simulink model "Controlled_simulink_model_vectorized"  (R2017b)
settings: Solver=VariableStepAuto  StartTime=0  StopTime=57  FixedStep=0.001  MaxStep=1e-4  MinStep=1e-5  RelTol=1e-5
values from neighbouring files (symbols this model uses):
  Accel_bias = 0    [Controlled_model_vectorized.m]
  Ax = 0.0    (= 0)    [Controlled_model_vectorized.m]
  Ay = 0.0    (= 0)    [Controlled_model_vectorized.m]
  Az = 0.0    (= 0)    [Controlled_model_vectorized.m]
  b = 1.144e-08    [Controlled_model_vectorized.m]
  b_m = 2.415e-6    (= 2.415e-06)    [Controlled_model_vectorized.m]
  d = 9.94e-10    [Controlled_model_vectorized.m]
  g = 9.81    [Controlled_model_vectorized.m]
  Gyro_bias = 0    [Controlled_model_vectorized.m]
  Ixx = 7.5*10^(-3)    (= 0.0075)    [Controlled_model_vectorized.m]
  Iyy = 7.5*10^(-3)    (= 0.0075)    [Controlled_model_vectorized.m]
  Izz = 1.3*10^(-2)    (= 0.013)    [Controlled_model_vectorized.m]
  Jr = 6.5*10^(-7)    (= 6.5e-07)    [Controlled_model_vectorized.m]
  Kemf = 0.00255    [Controlled_model_vectorized.m]
  Kt = Kemf    (= 0.00255)    [Controlled_model_vectorized.m]
  l = 0.23    [Controlled_model_vectorized.m]
  L = 0.001*R    (= 0.000117)    [Controlled_model_vectorized.m]
  m = weight/g    (= 0.0289500509684)    [Controlled_model_vectorized.m]
  R = 0.117    [Controlled_model_vectorized.m]
undefined symbols (not defined in the file or in its folder): sigbuilder_block
libraries: simulink x4
settings Model: Creator=Nicky  LastModifiedBy=Nicky
settings SolverCC: MaxConsecutiveMinStep=1000  ZeroCrossAlgorithm=Adaptive  AlgebraicLoopSolver=LineSearch  AutoInsertRateTranBlk=on
settings DebuggingCC: MaxConsecutiveZCsMsg=none
settings CodeAppCC: StateflowObjectComments=on
settings SimscapeCC: SimscapeNormalizeSystem=off

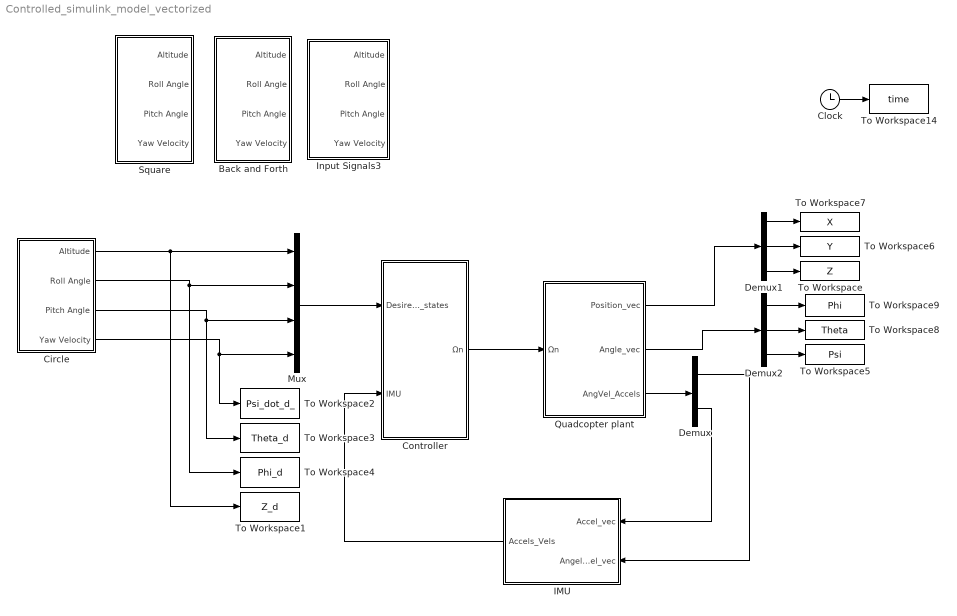
== system Controlled_simulink_model_vectorized ==
  Back and Forth : Subsystem  Tag=STV Subsys  LoadFcn=sigbuilder_block('load');  StartFcn=sigbuilder_block('start');  StopFcn=sigbuilder_block('stop');  ClipboardFcn=sigbuilder_block('clipboard');  mask(Sigbuilder block){tuvar=[0:10]}
      mask help: Simulink:masks:SigbuilderBlock_MD
      mask init:
      | if ~strcmp(get_param(bdroot(gcbh),'SimulationStatus'),'stopped') tuvar = sigbuilder_block('maskInit'); end
      settings: CopyFcn=sigbuilder_block('copy');  DeleteFcn=sigbuilder_block('delete');  ModelCloseFcn=sigbuilder_block('modelClose');  PreSaveFcn=sigbuilder_block('preSave');  PauseFcn=sigbuilder_block('pause');  ContinueFcn=sigbuilder_block('continue');  NameChangeFcn=sigbuilder_block('namechange');  OpenFcn=sigbuilder_block('open',[6 30 1428 682.5 ]);  CloseFcn=sigbuilder_block('close');
      mask Display: plot(0, 0, 100, 100,[2, 2, 32, 32, 2], [68, 8, 8, 68, 68],[32, 2], [38, 38], [32, 19, 2],[53, 60, 44], [32, 17, 17, 2],[16, 16, 31, 31]);txt = getActiveGroup(gcbh);text(2, 100, txt,'verticalAlignment', 'top');
  Circle : Subsystem  Tag=STV Subsys  LoadFcn=sigbuilder_block('load');  StartFcn=sigbuilder_block('start');  StopFcn=sigbuilder_block('stop');  ClipboardFcn=sigbuilder_block('clipboard');  mask(Sigbuilder block){tuvar=[0:10]}
      mask help: Simulink:masks:SigbuilderBlock_MD
      mask init:
      | if ~strcmp(get_param(bdroot(gcbh),'SimulationStatus'),'stopped') tuvar = sigbuilder_block('maskInit'); end
      settings: CopyFcn=sigbuilder_block('copy');  DeleteFcn=sigbuilder_block('delete');  ModelCloseFcn=sigbuilder_block('modelClose');  PreSaveFcn=sigbuilder_block('preSave');  PauseFcn=sigbuilder_block('pause');  ContinueFcn=sigbuilder_block('continue');  NameChangeFcn=sigbuilder_block('namechange');  OpenFcn=sigbuilder_block('open',[173.25 183.75 1012.5 456 ]);  CloseFcn=sigbuilder_block('close');
      mask Display: plot(0, 0, 100, 100,[2, 2, 32, 32, 2], [68, 8, 8, 68, 68],[32, 2], [38, 38], [32, 19, 2],[53, 60, 44], [32, 17, 17, 2],[16, 16, 31, 31]);txt = getActiveGroup(gcbh);text(2, 100, txt,'verticalAlignment', 'top');
  Clock : Clock
  Controller : Subsystem
  Demux : Demux  Outputs=2
  Demux1 : Demux  Outputs=3
  Demux2 : Demux  Outputs=3
  IMU : Subsystem
  Input Signals3 : Subsystem  Tag=STV Subsys  LoadFcn=sigbuilder_block('load');  StartFcn=sigbuilder_block('start');  StopFcn=sigbuilder_block('stop');  ClipboardFcn=sigbuilder_block('clipboard');  mask(Sigbuilder block){tuvar=[0:10]}
      mask help: Simulink:masks:SigbuilderBlock_MD
      mask init:
      | if ~strcmp(get_param(bdroot(gcbh),'SimulationStatus'),'stopped') tuvar = sigbuilder_block('maskInit'); end
      settings: CopyFcn=sigbuilder_block('copy');  DeleteFcn=sigbuilder_block('delete');  ModelCloseFcn=sigbuilder_block('modelClose');  PreSaveFcn=sigbuilder_block('preSave');  PauseFcn=sigbuilder_block('pause');  ContinueFcn=sigbuilder_block('continue');  NameChangeFcn=sigbuilder_block('namechange');  OpenFcn=sigbuilder_block('open',[6 46.5 1428 642 ]);  CloseFcn=sigbuilder_block('close');
      mask Display: plot(0, 0, 100, 100,[2, 2, 32, 32, 2], [68, 8, 8, 68, 68],[32, 2], [38, 38], [32, 19, 2],[53, 60, 44], [32, 17, 17, 2],[16, 16, 31, 31]);txt = getActiveGroup(gcbh);text(2, 100, txt,'verticalAlignment', 'top');
  Mux : Mux
  Quadcopter plant : Subsystem
  Square : Subsystem  Tag=STV Subsys  LoadFcn=sigbuilder_block('load');  StartFcn=sigbuilder_block('start');  StopFcn=sigbuilder_block('stop');  ClipboardFcn=sigbuilder_block('clipboard');  mask(Sigbuilder block){tuvar=[0:10]}
      mask help: Simulink:masks:SigbuilderBlock_MD
      mask init:
      | if ~strcmp(get_param(bdroot(gcbh),'SimulationStatus'),'stopped') tuvar = sigbuilder_block('maskInit'); end
      settings: CopyFcn=sigbuilder_block('copy');  DeleteFcn=sigbuilder_block('delete');  ModelCloseFcn=sigbuilder_block('modelClose');  PreSaveFcn=sigbuilder_block('preSave');  PauseFcn=sigbuilder_block('pause');  ContinueFcn=sigbuilder_block('continue');  NameChangeFcn=sigbuilder_block('namechange');  OpenFcn=sigbuilder_block('open',[6 30 1428 682.5 ]);  CloseFcn=sigbuilder_block('close');
      mask Display: plot(0, 0, 100, 100,[2, 2, 32, 32, 2], [68, 8, 8, 68, 68],[32, 2], [38, 38], [32, 19, 2],[53, 60, 44], [32, 17, 17, 2],[16, 16, 31, 31]);txt = getActiveGroup(gcbh);text(2, 100, txt,'verticalAlignment', 'top');
  To Workspace : ToWorkspace  VariableName=Z  SampleTime=0.001
      settings: Save2DSignal=2-D array (concatenate along first dimension)
  To Workspace1 : ToWorkspace  VariableName=Z_d  SampleTime=0.001
      settings: Save2DSignal=2-D array (concatenate along first dimension)
  To Workspace14 : ToWorkspace  VariableName=time  SampleTime=0.001
      settings: Save2DSignal=2-D array (concatenate along first dimension)
  To Workspace2 : ToWorkspace  VariableName=Psi_dot_d_  SampleTime=0.001
      settings: Save2DSignal=2-D array (concatenate along first dimension)
  To Workspace3 : ToWorkspace  VariableName=Theta_d  SampleTime=0.001
      settings: Save2DSignal=2-D array (concatenate along first dimension)
  To Workspace4 : ToWorkspace  VariableName=Phi_d  SampleTime=0.001
      settings: Save2DSignal=2-D array (concatenate along first dimension)
  To Workspace5 : ToWorkspace  VariableName=Psi  SampleTime=0.001
      settings: Save2DSignal=2-D array (concatenate along first dimension)
  To Workspace6 : ToWorkspace  VariableName=Y  SampleTime=0.001
      settings: Save2DSignal=2-D array (concatenate along first dimension)
  To Workspace7 : ToWorkspace  VariableName=X  SampleTime=0.001
      settings: Save2DSignal=2-D array (concatenate along first dimension)
  To Workspace8 : ToWorkspace  VariableName=Theta  SampleTime=0.001
      settings: Save2DSignal=2-D array (concatenate along first dimension)
  To Workspace9 : ToWorkspace  VariableName=Phi  SampleTime=0.001
      settings: Save2DSignal=2-D array (concatenate along first dimension)
  wires:
  Clock/1 -> To Workspace14/1
  Circle/4(Yaw Velocity) -> To Workspace2/1, Mux/4
  Circle/1(Altitude) -> To Workspace1/1, Mux/1
  Circle/3(Pitch Angle) -> To Workspace3/1, Mux/3
  Quadcopter plant/3(AngVel_Accels) -> Demux/1
  Controller/1(Ωn) -> Quadcopter plant/1(Ωn)
  Mux/1 -> Controller/1(Desired_states)
  IMU/1(Accels_Vels) -> Controller/2("IMU ")
  Quadcopter plant/1(Position_vec) -> Demux1/1
  Demux1/1 -> To Workspace7/1
  Demux1/2 -> To Workspace6/1
  Demux1/3 -> To Workspace/1
  Quadcopter plant/2(Angle_vec) -> Demux2/1
  Demux2/1 -> To Workspace9/1
  Demux2/2 -> To Workspace8/1
  Demux2/3 -> To Workspace5/1
  Demux/2 -> IMU/1(Accel_vec)
  Demux/1 -> IMU/2(Angel_vel_vec)
  Circle/2(Roll Angle) -> To Workspace4/1, Mux/2

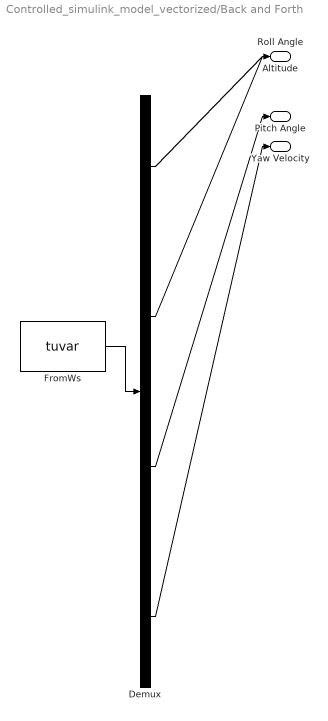
== system Controlled_simulink_model_vectorized/Back and Forth ==
  Demux : Demux  Tag=STV Demux
  FromWs : FromWorkspace  Tag=STV FromWs  VariableName=tuvar  SampleTime=0
      SigBuilderData=|
      | common.afterFinalStr = 'Extrapolate'
      | common.sampleTime = 0
      | dataSet.timeRange = [0 150]
      | dataSet.name = 'Group 1'
      | sbobj.Groups.Name = 'Group 1'
      | sbobj.Groups.Signals(1).Name = 'Altitude'
      | sbobj.Groups.Signals(1).XData = [0 1 150]
      | sbobj.Groups.Signals(1).YData = [0 1 5]
      | sbobj.Groups.Signals(2).Name = 'Roll Angle'
      | sbobj.Groups.Signals(2).XData = [0 5 6 8 9 18 19 21 22 31 32 34 35 44 45 47 48 57 150]
      | sbobj.Groups.Signals(2).YData = [0 0 -0.25 -0.25 0 0 0.25 0.25 0 0 -0.25 -0.25 0 0 0.25 0.25 0 0 0]
      | sbobj.Groups.Signals(3).Name = 'Pitch Angle'
      | sbobj.Groups.Signals(3).XData = [0 49 150]
      | sbobj.Groups.Signals(3).YData = [0 0 0]
      | sbobj.Groups.Signals(4).Name = 'Yaw Velocity'
      | sbobj.Groups.Signals(4).XData = [0 150]
      | sbobj.Groups.Signals(4).YData = [0 0]
      | sbobj.Groups.TimeRange = [0 150]
  Altitude : Outport  Tag=STV Outport
  Roll Angle : Outport  Tag=STV Outport  Port=2
  Pitch Angle : Outport  Tag=STV Outport  Port=3
  Yaw Velocity : Outport  Tag=STV Outport  Port=4
  wires:
  FromWs/1 -> Demux/1
  Demux/1 -> Altitude/1
  Demux/2 -> Roll Angle/1
  Demux/3 -> Pitch Angle/1
  Demux/4 -> Yaw Velocity/1

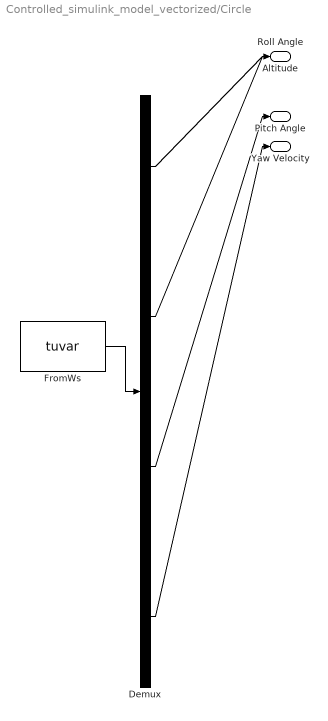
== system Controlled_simulink_model_vectorized/Circle ==
  Demux : Demux  Tag=STV Demux
  FromWs : FromWorkspace  Tag=STV FromWs  VariableName=tuvar  SampleTime=0
      SigBuilderData=|
      | common.afterFinalStr = 'Extrapolate'
      | common.sampleTime = 0
      | dataSet.timeRange = [0 150]
      | dataSet.name = 'Group 1'
      | sbobj.Groups.Name = 'Group 1'
      | sbobj.Groups.Signals(1).Name = 'Altitude'
      | sbobj.Groups.Signals(1).XData = [0 1 150]
      | sbobj.Groups.Signals(1).YData = [0 -1 -5]
      | sbobj.Groups.Signals(2).Name = 'Roll Angle'
      | sbobj.Groups.Signals(2).XData = [0 13 14 18 20 29 31 40 42 51 53 62 64 73 75 84 86 95 97 106 108 117 119 128 130 139 141 150]
      | sbobj.Groups.Signals(2).YData = [0 0 -0.1 -0.1 0.1 0.1 -0.1 -0.1 0.1 0.1 -0.1 -0.1 0.1 0.1 -0.1 -0.1 0.1 0.1 -0.1 -0.1 0.1 0.1 -0.1 -0.1 0.1 0.1 -0.1 -0.1]
      | sbobj.Groups.Signals(3).Name = 'Pitch Angle'
      | sbobj.Groups.Signals(3).XData = [0 7 8 12 14 23 25 34 36 45 47 56 58 67 69 78 80 89 91 100 102 111 113 122 124 133 135 144 146 150]
      | sbobj.Groups.Signals(3).YData = [0 0 -0.1 -0.1 0.1 0.1 -0.1 -0.1 0.1 0.1 -0.1 -0.1 0.1 0.1 -0.1 -0.1 0.1 0.1 -0.1 -0.1 0.1 0.1 -0.1 -0.1 0.1 0.1 -0.1 -0.1 0 0]
      | sbobj.Groups.Signals(4).Name = 'Yaw Velocity'
      | sbobj.Groups.Signals(4).XData = [0 150]
      | sbobj.Groups.Signals(4).YData = [0 0]
      | sbobj.Groups.TimeRange = [0 150]
  Altitude : Outport  Tag=STV Outport
  Roll Angle : Outport  Tag=STV Outport  Port=2
  Pitch Angle : Outport  Tag=STV Outport  Port=3
  Yaw Velocity : Outport  Tag=STV Outport  Port=4
  wires:
  FromWs/1 -> Demux/1
  Demux/1 -> Altitude/1
  Demux/2 -> Roll Angle/1
  Demux/3 -> Pitch Angle/1
  Demux/4 -> Yaw Velocity/1

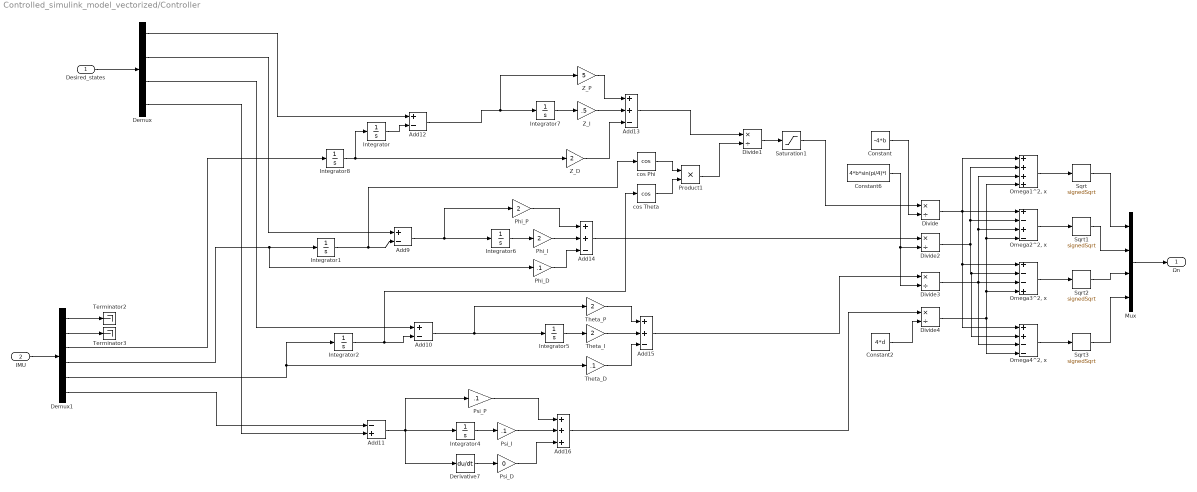
== system Controlled_simulink_model_vectorized/Controller ==
  Desired_states : Inport
  "IMU " : Inport  Port=2
  Add10 : Sum  Inputs=+-
  Add11 : Sum  Inputs=-+
  Add12 : Sum  Inputs=+-
  Add13 : Sum  Inputs=++-
  Add14 : Sum  Inputs=++-
  Add15 : Sum  Inputs=++-
  Add16 : Sum  Inputs=+++
  Add9 : Sum  Inputs=+-
  Constant : Constant  Value=-4*b
  Constant2 : Constant  Value=4*d
  Constant6 : Constant  Value=4*b*sin(pi/4)*l
  Demux : Demux
  Demux1 : Demux  Outputs=6
  Derivative7 : Derivative
  Divide{,1..4} (5 alike) : Product  Inputs=*/
  Integrator : Integrator  LimitOutput=on  UpperSaturationLimit=0
  Integrator1 : Integrator  WrapState=on
  Integrator2 : Integrator  WrapState=on
  Integrator{4..8} (5 alike) : Integrator
  Mux : Mux
  "Omega1^2, x" : Sum  Inputs=++++
  "Omega2^2, x" : Sum  Inputs=+-+-
  "Omega3^2, x" : Sum  Inputs=+--+
  "Omega4^2, x" : Sum  Inputs=++--
  Phi_D : Gain  Gain=.1
  Phi_I : Gain  Gain=2
  Phi_P : Gain  Gain=2
  Product1 : Product  RndMeth=Zero
  Psi_D : Gain  Gain=0
  Psi_I : Gain  Gain=.1
  Psi_P : Gain  Gain=.1
  Saturation1 : Saturate  UpperLimit=0  LowerLimit=-inf
  Sqrt{,1..3} (4 alike) : Sqrt  Operator=signedSqrt  SaturateOnIntegerOverflow=on
  Terminator2 : Terminator
  Terminator3 : Terminator
  Theta_D : Gain  Gain=.1
  Theta_I : Gain  Gain=2
  Theta_P : Gain  Gain=2
  Z_D : Gain  Gain=2
  "Z_I " : Gain  Gain=.5
  Z_P : Gain  Gain=5
  cos Phi : Trigonometry  Operator=cos
  cos Theta : Trigonometry  Operator=cos
  Ωn : Outport
  wires:
  Z_D/1 -> Add13/3
  Theta_I/1 -> Add15/2
  Add12/1 -> Z_P/1, Integrator7/1
  Add11/1 -> Derivative7/1, Integrator4/1, Psi_P/1
  "Z_I "/1 -> Add13/2
  Theta_P/1 -> Add15/1
  Integrator4/1 -> Psi_I/1
  Integrator7/1 -> "Z_I "/1
  Add9/1 -> Integrator6/1, Phi_P/1
  Derivative7/1 -> Psi_D/1
  Psi_D/1 -> Add16/3
  Psi_I/1 -> Add16/2
  Integrator6/1 -> Phi_I/1
  cos Theta/1 -> Product1/2
  Add13/1 -> Divide1/1
  Phi_D/1 -> Add14/3
  cos Phi/1 -> Product1/1
  Divide1/1 -> Saturation1/1
  Theta_D/1 -> Add15/3
  Integrator5/1 -> Theta_I/1
  Add10/1 -> Theta_P/1, Integrator5/1
  Product1/1 -> Divide1/2
  Phi_I/1 -> Add14/2
  Phi_P/1 -> Add14/1
  Psi_P/1 -> Add16/1
  Z_P/1 -> Add13/1
  Constant6/1 -> Divide3/2, Divide2/2
  Add14/1 -> Divide2/1
  Add15/1 -> Divide3/1
  Saturation1/1 -> Divide/1
  Constant/1 -> Divide/2
  Constant2/1 -> Divide4/2
  Add16/1 -> Divide4/1
  Divide4/1 -> "Omega3^2, x"/4, "Omega2^2, x"/4, "Omega1^2, x"/4, "Omega4^2, x"/4
  Divide2/1 -> "Omega4^2, x"/2, "Omega3^2, x"/2, "Omega2^2, x"/2, "Omega1^2, x"/2
  Divide3/1 -> "Omega4^2, x"/3, "Omega3^2, x"/3, "Omega2^2, x"/3, "Omega1^2, x"/3
  Divide/1 -> "Omega4^2, x"/1, "Omega3^2, x"/1, "Omega2^2, x"/1, "Omega1^2, x"/1
  "Omega1^2, x"/1 -> Sqrt/1
  "Omega2^2, x"/1 -> Sqrt1/1
  "Omega3^2, x"/1 -> Sqrt2/1
  "Omega4^2, x"/1 -> Sqrt3/1
  Integrator1/1 -> cos Phi/1, Add9/2
  Integrator2/1 -> cos Theta/1, Add10/2
  Integrator/1 -> Add12/2
  Integrator8/1 -> Z_D/1, Integrator/1
  Sqrt/1 -> Mux/1
  Sqrt1/1 -> Mux/2
  Sqrt2/1 -> Mux/3
  Sqrt3/1 -> Mux/4
  Mux/1 -> Ωn/1
  Desired_states/1 -> Demux/1
  "IMU "/1 -> Demux1/1
  Demux1/1 -> Terminator2/1
  Demux1/2 -> Terminator3/1
  Demux/1 -> Add12/1
  Demux/2 -> Add9/1
  Demux/3 -> Add10/1
  Demux/4 -> Add11/2
  Demux1/3 -> Integrator8/1
  Demux1/4 -> Phi_D/1, Integrator1/1
  Demux1/5 -> Integrator2/1, Theta_D/1
  Demux1/6 -> Add11/1

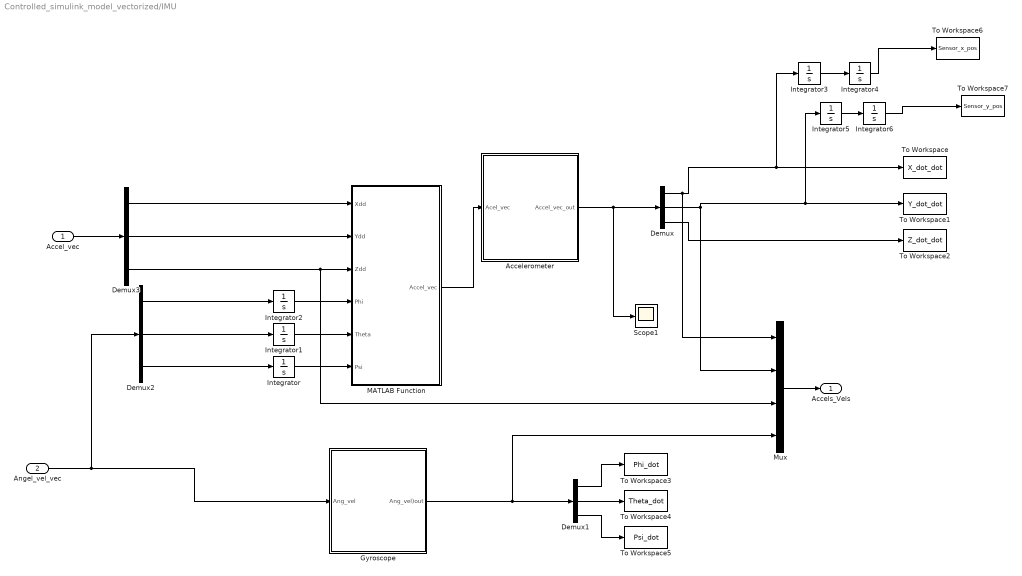
== system Controlled_simulink_model_vectorized/IMU ==
  Accel_vec : Inport
  Angel_vel_vec : Inport  Port=2
  Accelerometer : Subsystem
  Demux{,1..3} (4 alike) : Demux  Outputs=3
  Gyroscope : Subsystem
  Integrator{,3..6} (5 alike) : Integrator
  Integrator1 : Integrator  WrapState=on
  Integrator2 : Integrator  WrapState=on
  MATLAB Function : MATLAB Function  TreatAsAtomicUnit=on
  Mux : Mux
  Scope1 : Scope
  To Workspace : ToWorkspace  VariableName=X_dot_dot  SampleTime=0.001
      settings: Save2DSignal=2-D array (concatenate along first dimension)
  To Workspace1 : ToWorkspace  VariableName=Y_dot_dot  SampleTime=0.001
      settings: Save2DSignal=2-D array (concatenate along first dimension)
  To Workspace2 : ToWorkspace  VariableName=Z_dot_dot  SampleTime=0.001
      settings: Save2DSignal=2-D array (concatenate along first dimension)
  To Workspace3 : ToWorkspace  VariableName=Phi_dot  SampleTime=0.001
      settings: Save2DSignal=2-D array (concatenate along first dimension)
  To Workspace4 : ToWorkspace  VariableName=Theta_dot  SampleTime=0.001
      settings: Save2DSignal=2-D array (concatenate along first dimension)
  To Workspace5 : ToWorkspace  VariableName=Psi_dot  SampleTime=0.001
      settings: Save2DSignal=2-D array (concatenate along first dimension)
  To Workspace6 : ToWorkspace  VariableName=Sensor_x_pos  SampleTime=0.001
      settings: Save2DSignal=2-D array (concatenate along first dimension)
  To Workspace7 : ToWorkspace  VariableName=Sensor_y_pos  SampleTime=0.001
      settings: Save2DSignal=2-D array (concatenate along first dimension)
  Accels_Vels : Outport
  wires:
  MATLAB Function/1(Accel_vec) -> Accelerometer/1(Acel_vec)
  Demux/2 -> Mux/2, Integrator5/1, To Workspace1/1
  Demux/1 -> Mux/1, Integrator3/1, To Workspace/1
  Demux/3 -> To Workspace2/1
  Accelerometer/1(Accel_vec_out) -> Scope1/1, Demux/1
  Demux1/1 -> To Workspace3/1
  Gyroscope/1(Ang_vel)out) -> Mux/4, Demux1/1
  Demux1/2 -> To Workspace4/1
  Demux1/3 -> To Workspace5/1
  Angel_vel_vec/1 -> Demux2/1, Gyroscope/1(Ang_vel)
  Integrator/1 -> MATLAB Function/6(Psi)
  Integrator1/1 -> MATLAB Function/5(Theta)
  Integrator2/1 -> MATLAB Function/4(Phi)
  Demux2/3 -> Integrator/1
  Demux2/2 -> Integrator1/1
  Demux2/1 -> Integrator2/1
  Accel_vec/1 -> Demux3/1
  Demux3/1 -> MATLAB Function/1(Xdd)
  Demux3/2 -> MATLAB Function/2(Ydd)
  Demux3/3 -> Mux/3, MATLAB Function/3(Zdd)
  Mux/1 -> Accels_Vels/1
  Integrator3/1 -> Integrator4/1
  Integrator5/1 -> Integrator6/1
  Integrator4/1 -> To Workspace6/1
  Integrator6/1 -> To Workspace7/1

== system Controlled_simulink_model_vectorized/Input Signals3 ==
  Demux : Demux  Tag=STV Demux
  FromWs : FromWorkspace  Tag=STV FromWs  VariableName=tuvar  SampleTime=0
      SigBuilderData=|
      | common.afterFinalStr = 'Extrapolate'
      | common.sampleTime = 0
      | dataSet.timeRange = [0 150]
      | dataSet.name = 'Group 1'
      | sbobj.Groups.Name = 'Group 1'
      | sbobj.Groups.Signals(1).Name = 'Altitude'
      | sbobj.Groups.Signals(1).XData = [0 1 150]
      | sbobj.Groups.Signals(1).YData = [0 1 5]
      | sbobj.Groups.Signals(2).Name = 'Roll Angle'
      | sbobj.Groups.Signals(2).XData = [0 7 8 10 12 17 19 24 26 31 33 38 40 45 47 52 53 150]
      | sbobj.Groups.Signals(2).YData = [0 0 -0.25 -0.25 0.25 0.25 -0.25 -0.25 0.25 0.25 -0.25 -0.25 0.25 0.25 -0.25 -0.25 0 0]
      | sbobj.Groups.Signals(3).Name = 'Pitch Angle'
      | sbobj.Groups.Signals(3).XData = [0 3 4 6 8 13 15 20 22 27 29 29 34 36 41 43 48 49 150]
      | sbobj.Groups.Signals(3).YData = [0 0 -0.25 -0.25 0.25 0.25 -0.25 -0.25 0.25 0.25 -0.245 -0.25 -0.25 0.25 0.25 -0.25 -0.25 0 0]
      | sbobj.Groups.Signals(4).Name = 'Yaw Velocity'
      | sbobj.Groups.Signals(4).XData = [0 150]
      | sbobj.Groups.Signals(4).YData = [0 0]
      | sbobj.Groups.TimeRange = [0 150]
  Altitude : Outport  Tag=STV Outport
  Roll Angle : Outport  Tag=STV Outport  Port=2
  Pitch Angle : Outport  Tag=STV Outport  Port=3
  Yaw Velocity : Outport  Tag=STV Outport  Port=4
  wires:
  FromWs/1 -> Demux/1
  Demux/1 -> Altitude/1
  Demux/2 -> Roll Angle/1
  Demux/3 -> Pitch Angle/1
  Demux/4 -> Yaw Velocity/1

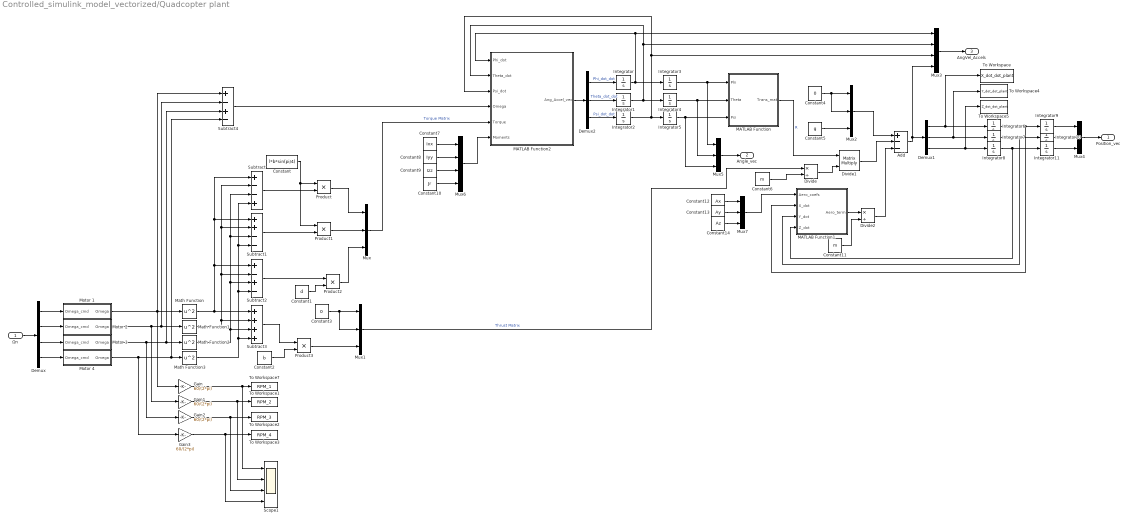
== system Controlled_simulink_model_vectorized/Quadcopter plant ==
  Ωn : Inport
  " Motor 1" : Subsystem
  " Motor 2" : Subsystem
  " Motor 3" : Subsystem
  " Motor 4" : Subsystem
  Add : Sum  Inputs=+--
  Constant : Constant  Value=l*b*sin(pi/4)
  Constant1 : Constant  Value=d
  Constant10 : Constant  Value=Jr
  Constant11 : Constant  Value=m
  Constant12 : Constant  Value=Ax
  Constant13 : Constant  Value=Ay
  Constant14 : Constant  Value=Az
  Constant2 : Constant  Value=b
  Constant3 : Constant  Value=0
  Constant4 : Constant  Value=0
  Constant5 : Constant  Value=g
  Constant6 : Constant  Value=m
  Constant7 : Constant  Value=Ixx
  Constant8 : Constant  Value=Iyy
  Constant9 : Constant  Value=Izz
  Demux : Demux
  Demux1 : Demux  Outputs=3
  Demux2 : Demux  Outputs=3
  Divide : Product  Inputs=*/
  Divide1 : Product  Inputs=**  Multiplication=Matrix(*)
  Divide2 : Product  Inputs=*/
  Gain{,1..3} (4 alike) : Gain  Gain=60/(2*pi)
  Integrator{,1..2,5..7,9..10} (8 alike) : Integrator
  Integrator11 : Integrator  LimitOutput=on  UpperSaturationLimit=0
  Integrator3 : Integrator  WrapState=on
  Integrator4 : Integrator  WrapState=on
  Integrator8 : Integrator  LowerSaturationLimit=0
  MATLAB Function : MATLAB Function  TreatAsAtomicUnit=on
  MATLAB Function1 : MATLAB Function  TreatAsAtomicUnit=on
  MATLAB Function2 : MATLAB Function  TreatAsAtomicUnit=on
  Math Function{,1..3} (4 alike) : Math  Operator=square  SaturateOnIntegerOverflow=on
  Mux{,1..2,4..5,7} (6 alike) : Mux  Inputs=3
  Mux3 : Mux
  Mux6 : Mux
  Product{,1..3} (4 alike) : Product
  Scope1 : Scope  NumInputPorts=4
  Subtract : Sum  Inputs=+--+
  Subtract1 : Sum  Inputs=++--
  Subtract2 : Sum  Inputs=+-+-
  Subtract3 : Sum  Inputs=++++
  Subtract4 : Sum  Inputs=+-+-
  To Workspace : ToWorkspace  VariableName=X_dot_dot_plant  SampleTime=0.001
      settings: Save2DSignal=2-D array (concatenate along first dimension)
  To Workspace1 : ToWorkspace  VariableName=RPM_2  SampleTime=0.001
      settings: Save2DSignal=2-D array (concatenate along first dimension)
  To Workspace2 : ToWorkspace  VariableName=RPM_3  SampleTime=0.001
      settings: Save2DSignal=2-D array (concatenate along first dimension)
  To Workspace3 : ToWorkspace  VariableName=RPM_4  SampleTime=0.001
      settings: Save2DSignal=2-D array (concatenate along first dimension)
  To Workspace4 : ToWorkspace  VariableName=Y_dot_dot_plant  SampleTime=0.001
      settings: Save2DSignal=2-D array (concatenate along first dimension)
  To Workspace5 : ToWorkspace  VariableName=Z_dot_dot_plant  SampleTime=0.001
      settings: Save2DSignal=2-D array (concatenate along first dimension)
  To Workspace7 : ToWorkspace  VariableName=RPM_1  SampleTime=0.001
      settings: Save2DSignal=2-D array (concatenate along first dimension)
  Position_vec : Outport
  Angle_vec : Outport  Port=2
  AngVel_Accels : Outport  Port=3
  wires:
  Ωn/1 -> Demux/1
  Demux/1 -> " Motor 1"/1(Omega_cmd)
  Demux/4 -> " Motor 4"/1(Omega_cmd)
  Demux/3 -> " Motor 3"/1(Omega_cmd)
  Demux/2 -> " Motor 2"/1(Omega_cmd)
  Constant/1 -> Product1/1, Product/1
  Subtract/1 -> Product/2
  Subtract1/1 -> Product1/2
  Subtract2/1 -> Product2/1
  Constant1/1 -> Product2/2
  Product1/1 -> Mux/2
  Product/1 -> Mux/1
  Product2/1 -> Mux/3
  Mux/1 -> MATLAB Function2/5(Torque)  "Torque Matrix"
  Subtract3/1 -> Product3/1
  Constant2/1 -> Product3/2
  Constant3/1 -> Mux1/2, Mux1/1
  Product3/1 -> Mux1/3
  Mux1/1 -> Divide/1  "Thrust Matrix"
  Math Function/1 -> Subtract3/1, Subtract2/1, Subtract1/1, Subtract/1
  Math Function1/1 -> Subtract2/2, Subtract1/2, Subtract/2, Subtract3/2
  Math Function3/1 -> Subtract3/4, Subtract2/4, Subtract1/4, Subtract/4
  Math Function2/1 -> Subtract3/3, Subtract2/3, Subtract1/3, Subtract/3
  Constant4/1 -> Mux2/2, Mux2/1
  Constant5/1 -> Mux2/3
  Constant6/1 -> Divide/2
  Divide/1 -> Divide1/2
  MATLAB Function/1(Trans_mat) -> Divide1/1  "R"
  Mux2/1 -> Add/1
  Divide1/1 -> Add/2
  Add/1 -> Demux1/1, Mux3/4
  Subtract4/1 -> MATLAB Function2/4(Omega)
  MATLAB Function2/1(Ang_Accel_vec) -> Demux2/1
  Demux2/1 -> Integrator/1  "Phi_dot_dot"
  Demux2/2 -> Integrator1/1  "Theta_dot_dot"
  Demux2/3 -> Integrator2/1  "Psi_dot_dot"
  Integrator/1 -> Integrator3/1, MATLAB Function2/1(Phi_dot), Mux3/1
  Integrator1/1 -> Integrator4/1, MATLAB Function2/2(Theta_dot), Mux3/2
  Integrator2/1 -> Integrator5/1, MATLAB Function2/3(Psi_dot), Mux3/3
  Integrator3/1 -> Mux5/1, MATLAB Function/1(Phi)
  Integrator4/1 -> Mux5/2, MATLAB Function/2(Theta)
  Integrator5/1 -> Mux5/3, MATLAB Function/3(Psi)
  Mux3/1 -> AngVel_Accels/1
  Demux1/1 -> To Workspace/1, Integrator6/1
  Demux1/2 -> To Workspace4/1, Integrator7/1
  Demux1/3 -> To Workspace5/1, Integrator8/1
  Integrator7/1 -> Integrator10/1, MATLAB Function1/3(Y_dot)
  Integrator6/1 -> Integrator9/1, MATLAB Function1/2(X_dot)
  Integrator8/1 -> Integrator11/1, MATLAB Function1/4(Z_dot)
  Integrator9/1 -> Mux4/1
  Integrator10/1 -> Mux4/2
  Integrator11/1 -> Mux4/3
  Mux4/1 -> Position_vec/1
  Mux5/1 -> Angle_vec/1
  Constant7/1 -> Mux6/1
  Constant8/1 -> Mux6/2
  Constant9/1 -> Mux6/3
  Mux6/1 -> MATLAB Function2/6(Moments)
  Constant10/1 -> Mux6/4
  " Motor 1"/1(Omega) -> Gain/1, Subtract4/1, Math Function/1
  " Motor 2"/1(Omega) -> Gain1/1, Subtract4/2, Math Function1/1
  " Motor 3"/1(Omega) -> Gain2/1, Subtract4/3, Math Function2/1
  " Motor 4"/1(Omega) -> Gain3/1, Subtract4/4, Math Function3/1
  Gain/1 -> Scope1/1, To Workspace7/1
  Gain1/1 -> Scope1/2, To Workspace1/1
  Gain2/1 -> Scope1/3, To Workspace2/1
  Gain3/1 -> Scope1/4, To Workspace3/1
  Constant11/1 -> Divide2/2
  MATLAB Function1/1(Aero_term) -> Divide2/1
  Divide2/1 -> Add/3
  Constant12/1 -> Mux7/1
  Constant13/1 -> Mux7/2
  Constant14/1 -> Mux7/3
  Mux7/1 -> MATLAB Function1/1(Aero_coefs)

== system Controlled_simulink_model_vectorized/Square ==
  Demux : Demux  Tag=STV Demux
  FromWs : FromWorkspace  Tag=STV FromWs  VariableName=tuvar  SampleTime=0
      SigBuilderData=|
      | common.afterFinalStr = 'Extrapolate'
      | common.sampleTime = 0
      | dataSet.timeRange = [0 150]
      | dataSet.name = 'Group 1'
      | sbobj.Groups.Name = 'Group 1'
      | sbobj.Groups.Signals(1).Name = 'Altitude'
      | sbobj.Groups.Signals(1).XData = [0 1.04 60 60 150]
      | sbobj.Groups.Signals(1).YData = [1 1 1 2 2]
      | sbobj.Groups.Signals(2).Name = 'Roll Angle'
      | sbobj.Groups.Signals(2).XData = [0 2 3 5 6 8 9 11 12 30 31 33 34 36 37 39 40 75 76 78 79 81 82 84 85 103 104 106 107 109 110 112 113 150]
      | sbobj.Groups.Signals(2).YData = [0 0 0.2 0.2 0 0 -0.2 -0.2 0 0 -0.2 -0.2 0 0 0.2 0.2 0 0 0.2 0.2 0 0 -0.2 -0.2 0 0 -0.2 -0.2 0 0 0.2 0.2 0 0]
      | sbobj.Groups.Signals(3).Name = 'Pitch Angle'
      | sbobj.Groups.Signals(3).XData = [0 16 17 19 20 22 23 25 26 44 45 47 48 50 51 53 54 89 90 92 93 95 96 98 99 117 117 118 120 121 123 124 126 127 140.4 150]
      | sbobj.Groups.Signals(3).YData = [0 0 0.2 0.2 0 0 -0.2 -0.2 0 0 -0.2 -0.2 0 0 0.2 0.2 0 0 0.2 0.2 0 0 -0.2 -0.2 0 0 0.005 -0.2 -0.2 0 0 0.2 0.2 0 0 0]
      | sbobj.Groups.Signals(4).Name = 'Yaw Velocity'
      | sbobj.Groups.Signals(4).XData = [0 65 66 70 71 150]
      | sbobj.Groups.Signals(4).YData = [0 0 0.5 0.5 0 0]
      | sbobj.Groups.TimeRange = [0 150]
  Altitude : Outport  Tag=STV Outport
  Roll Angle : Outport  Tag=STV Outport  Port=2
  Pitch Angle : Outport  Tag=STV Outport  Port=3
  Yaw Velocity : Outport  Tag=STV Outport  Port=4
  wires:
  FromWs/1 -> Demux/1
  Demux/1 -> Altitude/1
  Demux/2 -> Roll Angle/1
  Demux/3 -> Pitch Angle/1
  Demux/4 -> Yaw Velocity/1

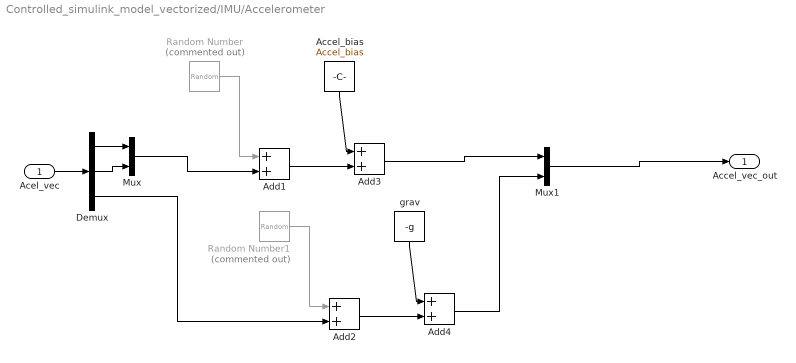
== system Controlled_simulink_model_vectorized/IMU/Accelerometer ==
  Acel_vec : Inport
  Accel_bias : Constant  Value=Accel_bias
  Add{1..4} (4 alike) : Sum
  Demux : Demux  Outputs=3
  Mux : Mux  Inputs=2
  Mux1 : Mux  Inputs=2
  Random Number : RandomNumber  Commented=on  Variance=0.0001  Seed=4  SampleTime=0.001
  Random Number1 : RandomNumber  Commented=on  Variance=0.0001  Seed=4  SampleTime=0.001
  grav : Constant  Value=-g
  Accel_vec_out : Outport
  wires:
  Accel_bias/1 -> Add3/1
  Add1/1 -> Add3/2
  Random Number/1 -> Add1/1
  Acel_vec/1 -> Demux/1
  Demux/1 -> Mux/1
  Demux/2 -> Mux/2
  Mux/1 -> Add1/2
  Add2/1 -> Add4/2
  Add4/1 -> Mux1/2
  grav/1 -> Add4/1
  Demux/3 -> Add2/2
  Random Number1/1 -> Add2/1
  Mux1/1 -> Accel_vec_out/1
  Add3/1 -> Mux1/1

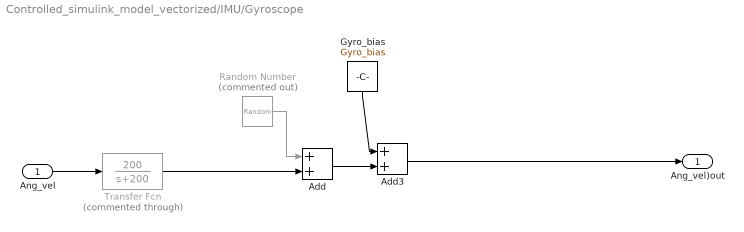
== system Controlled_simulink_model_vectorized/IMU/Gyroscope ==
  Ang_vel : Inport
  Add : Sum
  Add3 : Sum
  Gyro_bias : Constant  Value=Gyro_bias
  Random Number : RandomNumber  Commented=on  Variance=0.0001  Seed=4  SampleTime=0.001
  Transfer Fcn : TransferFcn  Commented=through  Numerator=[200]  Denominator=[1 200]
  Ang_vel)out : Outport
  wires:
  Ang_vel/1 -> Transfer Fcn/1
  Add/1 -> Add3/2
  Gyro_bias/1 -> Add3/1
  Random Number/1 -> Add/1
  Add3/1 -> Ang_vel)out/1
  Transfer Fcn/1 -> Add/2

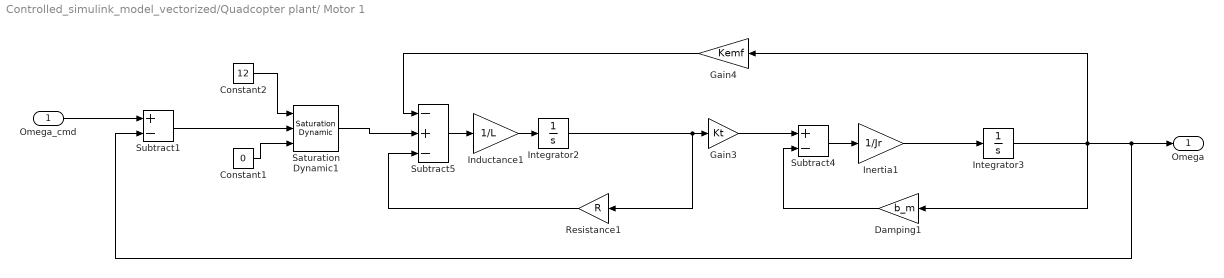
== system Controlled_simulink_model_vectorized/Quadcopter plant/ Motor 1 ==
  Omega_cmd : Inport
  Constant1 : Constant  Value=0
  Constant2 : Constant  Value=12
  Damping1 : Gain  Gain=b_m
  Gain3 : Gain  Gain=Kt
  Gain4 : Gain  Gain=Kemf
  Inductance1 : Gain  Gain=1/L
  Inertia1 : Gain  Gain=1/Jr
  Integrator2 : Integrator  LimitOutput=on  LowerSaturationLimit=0
  Integrator3 : Integrator  LimitOutput=on  LowerSaturationLimit=0
  Resistance1 : Gain  Gain=R
  Saturation Dynamic1 : simulink/Discontinuities/Saturation Dynamic  OutMin=[]  OutMax=[]  OutDataTypeStr=Inherit: Same as second input  OutDataType=fixdt(1, 16)  OutScaling=2^-10  DoSatur=off
  Subtract1 : Sum  Inputs=+-
  Subtract4 : Sum  Inputs=+-
  Subtract5 : Sum  Inputs=-+-
  Omega : Outport
  wires:
  Inductance1/1 -> Integrator2/1
  Inertia1/1 -> Integrator3/1
  Resistance1/1 -> Subtract5/3
  Damping1/1 -> Subtract4/2
  Subtract5/1 -> Inductance1/1
  Saturation Dynamic1/1 -> Subtract5/2
  Gain4/1 -> Subtract5/1
  Subtract4/1 -> Inertia1/1
  Gain3/1 -> Subtract4/1
  Omega_cmd/1 -> Subtract1/1
  Integrator3/1 -> Subtract1/2, Omega/1, Damping1/1, Gain4/1
  Constant1/1 -> Saturation Dynamic1/3
  Subtract1/1 -> Saturation Dynamic1/2
  Integrator2/1 -> Resistance1/1, Gain3/1
  Constant2/1 -> Saturation Dynamic1/1

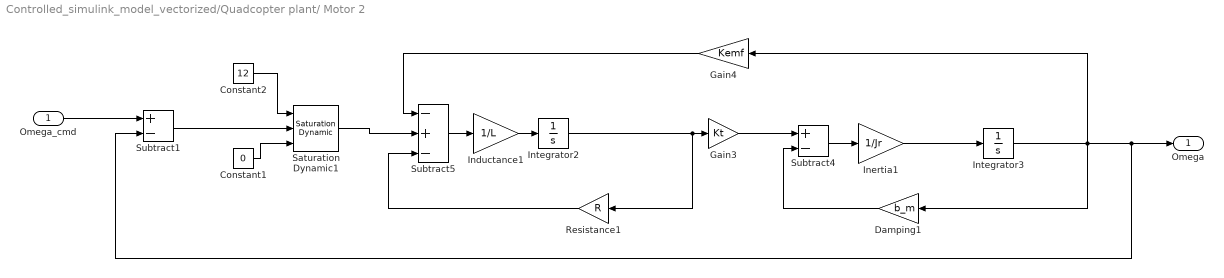
== system Controlled_simulink_model_vectorized/Quadcopter plant/ Motor 2 ==
  Omega_cmd : Inport
  Constant1 : Constant  Value=0
  Constant2 : Constant  Value=12
  Damping1 : Gain  Gain=b_m
  Gain3 : Gain  Gain=Kt
  Gain4 : Gain  Gain=Kemf
  Inductance1 : Gain  Gain=1/L
  Inertia1 : Gain  Gain=1/Jr
  Integrator2 : Integrator  LimitOutput=on  LowerSaturationLimit=0
  Integrator3 : Integrator  LimitOutput=on  LowerSaturationLimit=0
  Resistance1 : Gain  Gain=R
  Saturation Dynamic1 : simulink/Discontinuities/Saturation Dynamic  OutMin=[]  OutMax=[]  OutDataTypeStr=Inherit: Same as second input  OutDataType=fixdt(1, 16)  OutScaling=2^-10  DoSatur=off
  Subtract1 : Sum  Inputs=+-
  Subtract4 : Sum  Inputs=+-
  Subtract5 : Sum  Inputs=-+-
  Omega : Outport
  wires:
  Inductance1/1 -> Integrator2/1
  Inertia1/1 -> Integrator3/1
  Resistance1/1 -> Subtract5/3
  Damping1/1 -> Subtract4/2
  Subtract5/1 -> Inductance1/1
  Saturation Dynamic1/1 -> Subtract5/2
  Gain4/1 -> Subtract5/1
  Subtract4/1 -> Inertia1/1
  Gain3/1 -> Subtract4/1
  Omega_cmd/1 -> Subtract1/1
  Integrator3/1 -> Subtract1/2, Omega/1, Damping1/1, Gain4/1
  Constant1/1 -> Saturation Dynamic1/3
  Subtract1/1 -> Saturation Dynamic1/2
  Integrator2/1 -> Resistance1/1, Gain3/1
  Constant2/1 -> Saturation Dynamic1/1

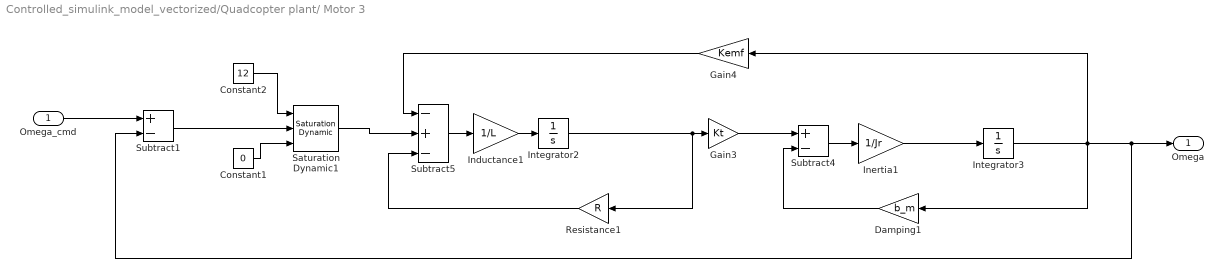
== system Controlled_simulink_model_vectorized/Quadcopter plant/ Motor 3 ==
  Omega_cmd : Inport
  Constant1 : Constant  Value=0
  Constant2 : Constant  Value=12
  Damping1 : Gain  Gain=b_m
  Gain3 : Gain  Gain=Kt
  Gain4 : Gain  Gain=Kemf
  Inductance1 : Gain  Gain=1/L
  Inertia1 : Gain  Gain=1/Jr
  Integrator2 : Integrator  LimitOutput=on  LowerSaturationLimit=0
  Integrator3 : Integrator  LimitOutput=on  LowerSaturationLimit=0
  Resistance1 : Gain  Gain=R
  Saturation Dynamic1 : simulink/Discontinuities/Saturation Dynamic  OutMin=[]  OutMax=[]  OutDataTypeStr=Inherit: Same as second input  OutDataType=fixdt(1, 16)  OutScaling=2^-10  DoSatur=off
  Subtract1 : Sum  Inputs=+-
  Subtract4 : Sum  Inputs=+-
  Subtract5 : Sum  Inputs=-+-
  Omega : Outport
  wires:
  Inductance1/1 -> Integrator2/1
  Inertia1/1 -> Integrator3/1
  Resistance1/1 -> Subtract5/3
  Damping1/1 -> Subtract4/2
  Subtract5/1 -> Inductance1/1
  Saturation Dynamic1/1 -> Subtract5/2
  Gain4/1 -> Subtract5/1
  Subtract4/1 -> Inertia1/1
  Gain3/1 -> Subtract4/1
  Omega_cmd/1 -> Subtract1/1
  Integrator3/1 -> Subtract1/2, Omega/1, Damping1/1, Gain4/1
  Constant1/1 -> Saturation Dynamic1/3
  Subtract1/1 -> Saturation Dynamic1/2
  Integrator2/1 -> Resistance1/1, Gain3/1
  Constant2/1 -> Saturation Dynamic1/1

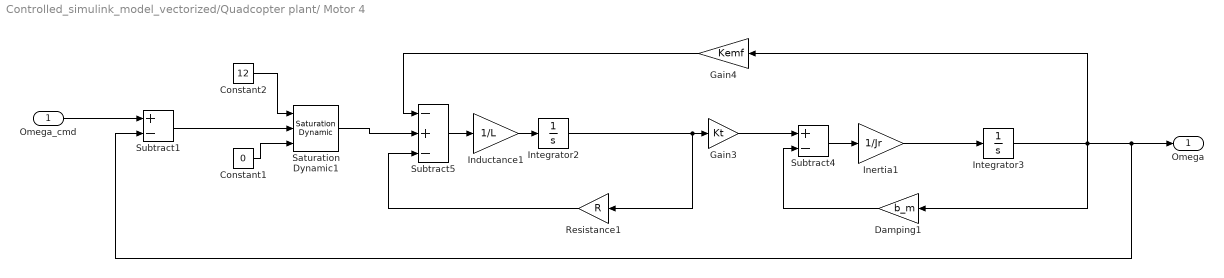
== system Controlled_simulink_model_vectorized/Quadcopter plant/ Motor 4 ==
  Omega_cmd : Inport
  Constant1 : Constant  Value=0
  Constant2 : Constant  Value=12
  Damping1 : Gain  Gain=b_m
  Gain3 : Gain  Gain=Kt
  Gain4 : Gain  Gain=Kemf
  Inductance1 : Gain  Gain=1/L
  Inertia1 : Gain  Gain=1/Jr
  Integrator2 : Integrator  LimitOutput=on  LowerSaturationLimit=0
  Integrator3 : Integrator  LimitOutput=on  LowerSaturationLimit=0
  Resistance1 : Gain  Gain=R
  Saturation Dynamic1 : simulink/Discontinuities/Saturation Dynamic  OutMin=[]  OutMax=[]  OutDataTypeStr=Inherit: Same as second input  OutDataType=fixdt(1, 16)  OutScaling=2^-10  DoSatur=off
  Subtract1 : Sum  Inputs=+-
  Subtract4 : Sum  Inputs=+-
  Subtract5 : Sum  Inputs=-+-
  Omega : Outport
  wires:
  Inductance1/1 -> Integrator2/1
  Inertia1/1 -> Integrator3/1
  Resistance1/1 -> Subtract5/3
  Damping1/1 -> Subtract4/2
  Subtract5/1 -> Inductance1/1
  Saturation Dynamic1/1 -> Subtract5/2
  Gain4/1 -> Subtract5/1
  Subtract4/1 -> Inertia1/1
  Gain3/1 -> Subtract4/1
  Omega_cmd/1 -> Subtract1/1
  Integrator3/1 -> Subtract1/2, Omega/1, Damping1/1, Gain4/1
  Constant1/1 -> Saturation Dynamic1/3
  Subtract1/1 -> Saturation Dynamic1/2
  Integrator2/1 -> Resistance1/1, Gain3/1
  Constant2/1 -> Saturation Dynamic1/1

== matlab function Controlled_simulink_model_vectorized/Quadcopter plant/MATLAB Function ==
  data: Trans_mat output; Phi input; Theta input; Psi input
function Trans_mat = Body2WorldAccels(Phi,Theta,Psi)
%XYZ
Trans_mat=[(cos(Psi)*cos(Theta)), (-sin(Psi)*cos(Phi)+cos(Psi)*sin(Theta)*sin(Phi)), (sin(Psi)*sin(Phi)+cos(Psi)*sin(Theta)*cos(Phi));...
          (sin(Psi)*cos(Theta)), (cos(Psi)*cos(Phi)+sin(Theta)*sin(Psi)*sin(Phi)), (-cos(Psi)*sin(Phi)+sin(Theta)*sin(Psi)*cos(Phi));...
          (-sin(Theta)), (cos(Theta)*sin(Phi)), (cos(Theta)*cos(Phi))];
      


R_Phi=[1, 0, 0;...
       0, cos(Phi), sin(Phi);...
       0, -sin(Phi), cos(Phi)];
   
R_Theta=[cos(Theta), 0, -sin(Theta);...
        0, 1, 0;...
        sin(Theta), 0, cos(Theta)];

R_Psi=[cos(Psi), sin(Psi), 0;...
       -sin(Psi), cos(Psi), 0;...
       0, 0, 1];
   
  Trans_mat= R_Psi*R_Theta*R_Phi;
  Trans_mat=Trans_mat;

== matlab function Controlled_simulink_model_vectorized/IMU/MATLAB Function ==
  data: Xdd input; Ydd input; Accel_vec output; Zdd input; Phi input; Theta input; Psi input
function Accel_vec = World2Body(Xdd,Ydd,Zdd,Phi,Theta,Psi)

Trans_mat=[(cos(Psi)*cos(Theta)), (-sin(Psi)*cos(Phi)+cos(Psi)*sin(Theta)*sin(Phi)), (sin(Psi)*sin(Phi)+cos(Psi)*sin(Theta)*cos(Phi));...
          (sin(Psi)*cos(Theta)), (cos(Psi)*cos(Phi)+sin(Theta)*sin(Psi)*sin(Phi)), (-cos(Psi)*sin(Phi)+sin(Theta)*sin(Psi)*cos(Phi));...
          (-sin(Theta)), (cos(Theta)*sin(Phi)), (cos(Theta)*cos(Phi))];
R_Phi=[1, 0, 0;...
       0, cos(Phi), sin(Phi);...
       0, -sin(Phi), cos(Phi)];
   
R_Theta=[cos(Theta), 0, -sin(Theta);...
        0, 1, 0;...
        sin(Theta), 0, cos(Theta)];

R_Psi=[cos(Psi), sin(Psi), 0;...
       -sin(Psi), cos(Psi), 0;...
       0, 0, 1];
   
 Trans_mat= R_Psi*R_Theta*R_Phi;

     

 

Accel_world=[Xdd;Ydd;Zdd];
Accel_vec=Trans_mat^-1*Accel_world;

== matlab function Controlled_simulink_model_vectorized/Quadcopter plant/MATLAB Function1 ==
  data: Aero_coefs input; Aero_term output; X_dot input; Y_dot input; Z_dot input
function Aero_term = Aero_Mat(Aero_coefs,X_dot,Y_dot,Z_dot)
Ax=Aero_coefs(1);
Ay=Aero_coefs(2);
Az=Aero_coefs(3);

A_mat=[Ax,0, 0;...
       0, Ay,0;...
       0, 0, Az];
Aero_term=A_mat*[X_dot;Y_dot;Z_dot];

== matlab function Controlled_simulink_model_vectorized/Quadcopter plant/MATLAB Function2 ==
  data: Phi_dot input; Ang_Accel_vec output; Theta_dot input; Psi_dot input; Omega input; Torque input; Moments input
function Ang_Accel_vec = Ang_Accel(Phi_dot,Theta_dot,Psi_dot,Omega,Torque,Moments)
Ixx=Moments(1);
Iyy=Moments(2);
Izz=Moments(3);
Jr=Moments(4);
Body_gyro_effect=[((Iyy-Izz)*Theta_dot*Psi_dot/Ixx);...
       ((Izz-Ixx)*Phi_dot*Psi_dot/Iyy);...
       ((Ixx-Iyy)*Phi_dot*Theta_dot/Izz)];
Rotor_inertia=[Theta_dot/Ixx;...
       -Phi_dot/Iyy;...
       0];
Actuator_action=[Torque(1)/Ixx;...
       Torque(2)/Iyy;...
       Torque(3)/Izz];
   
Ang_Accel_vec=Body_gyro_effect-(Jr.*Rotor_inertia.*Omega)+Actuator_action;
